simulink model "SAME5x_PIM_MCLV2_ioconfig"  (R2020b)
(part 2 of 3)

      mask TypeOptions CTXT4: Not Assigned | Alternate Register set assigned to IPL level 7 | Alternate Register set assigned to IPL level 6 | Alternate Register set assigned to IPL level 5 | Alternate Register set assigned to IPL level 4 | Alternate Register set assigned to IPL level 3 | Alternate Register set assigned to IPL level 2 | Alternate Register set assigned to IPL level 1
      mask TypeOptions MBXM0: Mailbox register configured for Master data read (Slave to Master data transfer) | Mailbox register configured for Master data write (Master to Slave data transfer)
      mask TypeOptions MBXM1: Mailbox register configured for Master data read (Slave to Master data transfer) | Mailbox register configured for Master data write (Master to Slave data transfer)
      mask TypeOptions MBXM2: Mailbox register configured for Master data read (Slave to Master data transfer) | Mailbox register configured for Master data write (Master to Slave data transfer)
      mask TypeOptions MBXM3: Mailbox register configured for Master data read (Slave to Master data transfer) | Mailbox register configured for Master data write (Master to Slave data transfer)
      mask TypeOptions MBXM4: Mailbox register configured for Master data read (Slave to Master data transfer) | Mailbox register configured for Master data write (Master to Slave data transfer)
      mask TypeOptions MBXM5: Mailbox register configured for Master data read (Slave to Master data transfer) | Mailbox register configured for Master data write (Master to Slave data transfer)
      mask TypeOptions MBXM6: Mailbox register configured for Master data read (Slave to Master data transfer) | Mailbox register configured for Master data write (Master to Slave data transfer)
      mask TypeOptions MBXM7: Mailbox register configured for Master data read (Slave to Master data transfer) | Mailbox register configured for Master data write (Master to Slave data transfer)
      mask TypeOptions MBXM8: Mailbox register configured for Master data read (Slave to Master data transfer) | Mailbox register configured for Master data write (Master to Slave data transfer)
      mask TypeOptions MBXM9: Mailbox register configured for Master data read (Slave to Master data transfer) | Mailbox register configured for Master data write (Master to Slave data transfer)
      mask TypeOptions MBXM10: Mailbox register configured for Master data read (Slave to Master data transfer) | Mailbox register configured for Master data write (Master to Slave data transfer)
      mask TypeOptions MBXM11: Mailbox register configured for Master data read (Slave to Master data transfer) | Mailbox register configured for Master data write (Master to Slave data transfer)
      mask TypeOptions MBXM12: Mailbox register configured for Master data read (Slave to Master data transfer) | Mailbox register configured for Master data write (Master to Slave data transfer)
      mask TypeOptions MBXM13: Mailbox register configured for Master data read (Slave to Master data transfer) | Mailbox register configured for Master data write (Master to Slave data transfer)
      mask TypeOptions MBXM14: Mailbox register configured for Master data read (Slave to Master data transfer) | Mailbox register configured for Master data write (Master to Slave data transfer)
      mask TypeOptions MBXM15: Mailbox register configured for Master data read (Slave to Master data transfer) | Mailbox register configured for Master data write (Master to Slave data transfer)
      mask TypeOptions MBXHSA: MSIxMBXD15 assigned to mailbox handshake protocol block A | MSIxMBXD14 assigned to mailbox handshake protocol block A | MSIxMBXD13 assigned to mailbox handshake protocol block A | MSIxMBXD12 assigned to mailbox handshake protocol block A | MSIxMBXD11 assigned to mailbox handshake protocol block A | MSIxMBXD10 assigned to mailbox handshake protocol block A | MSIxMBXD9 assigned to mailbox handshake protocol block A | MSIxMBXD8 assigned to mailbox handshake protocol block A | MSIxMBXD7 assigned to mailbox handshake protocol block A | MSIxMBXD6 assigned to mailbox handshake protocol block A | MSIxMBXD5 assigned to mailbox handshake protocol block A | MSIxMBXD4 assigned to mailbox handshake protocol block A | MSIxMBXD3 assigned to mailbox handshake protocol block A | MSIxMBXD2 assigned to mailbox handshake protocol block A | MSIxMBXD1 assigned to mailbox handshake protocol block A | MSIxMBXD0 assigned to mailbox handshake protocol block A
      mask TypeOptions MBXHSB: MSIxMBXD15 assigned to mailbox handshake protocol block B | MSIxMBXD14 assigned to mailbox handshake protocol block B | MSIxMBXD13 assigned to mailbox handshake protocol block B | MSIxMBXD12 assigned to mailbox handshake protocol block B | MSIxMBXD11 assigned to mailbox handshake protocol block B | MSIxMBXD10 assigned to mailbox handshake protocol block B | MSIxMBXD9 assigned to mailbox handshake protocol block B | MSIxMBXD8 assigned to mailbox handshake protocol block B | MSIxMBXD7 assigned to mailbox handshake protocol block B | MSIxMBXD6 assigned to mailbox handshake protocol block B | MSIxMBXD5 assigned to mailbox handshake protocol block B | MSIxMBXD4 assigned to mailbox handshake protocol block B | MSIxMBXD3 assigned to mailbox handshake protocol block B | MSIxMBXD2 assigned to mailbox handshake protocol block B | MSIxMBXD1 assigned to mailbox handshake protocol block B | MSIxMBXD0 assigned to mailbox handshake protocol block B
      mask TypeOptions MBXHSC: MSIxMBXD15 assigned to mailbox handshake protocol block C | MSIxMBXD14 assigned to mailbox handshake protocol block C | MSIxMBXD13 assigned to mailbox handshake protocol block C | MSIxMBXD12 assigned to mailbox handshake protocol block C | MSIxMBXD11 assigned to mailbox handshake protocol block C | MSIxMBXD10 assigned to mailbox handshake protocol block C | MSIxMBXD9 assigned to mailbox handshake protocol block C | MSIxMBXD8 assigned to mailbox handshake protocol block C | MSIxMBXD7 assigned to mailbox handshake protocol block C | MSIxMBXD6 assigned to mailbox handshake protocol block C | MSIxMBXD5 assigned to mailbox handshake protocol block C | MSIxMBXD4 assigned to mailbox handshake protocol block C | MSIxMBXD3 assigned to mailbox handshake protocol block C | MSIxMBXD2 assigned to mailbox handshake protocol block C | MSIxMBXD1 assigned to mailbox handshake protocol block C | MSIxMBXD0 assigned to mailbox handshake protocol block C
      mask TypeOptions MBXHSD: MSIxMBXD15 assigned to mailbox handshake protocol block D | MSIxMBXD14 assigned to mailbox handshake protocol block D | MSIxMBXD13 assigned to mailbox handshake protocol block D | MSIxMBXD12 assigned to mailbox handshake protocol block D | MSIxMBXD11 assigned to mailbox handshake protocol block D | MSIxMBXD10 assigned to mailbox handshake protocol block D | MSIxMBXD9 assigned to mailbox handshake protocol block D | MSIxMBXD8 assigned to mailbox handshake protocol block D | MSIxMBXD7 assigned to mailbox handshake protocol block D | MSIxMBXD6 assigned to mailbox handshake protocol block D | MSIxMBXD5 assigned to mailbox handshake protocol block D | MSIxMBXD4 assigned to mailbox handshake protocol block D | MSIxMBXD3 assigned to mailbox handshake protocol block D | MSIxMBXD2 assigned to mailbox handshake protocol block D | MSIxMBXD1 assigned to mailbox handshake protocol block D | MSIxMBXD0 assigned to mailbox handshake protocol block D
      mask TypeOptions MBXHSE: MSIxMBXD15 assigned to mailbox handshake protocol block E | MSIxMBXD14 assigned to mailbox handshake protocol block E | MSIxMBXD13 assigned to mailbox handshake protocol block E | MSIxMBXD12 assigned to mailbox handshake protocol block E | MSIxMBXD11 assigned to mailbox handshake protocol block E | MSIxMBXD10 assigned to mailbox handshake protocol block E | MSIxMBXD9 assigned to mailbox handshake protocol block E | MSIxMBXD8 assigned to mailbox handshake protocol block E | MSIxMBXD7 assigned to mailbox handshake protocol block E | MSIxMBXD6 assigned to mailbox handshake protocol block E | MSIxMBXD5 assigned to mailbox handshake protocol block E | MSIxMBXD4 assigned to mailbox handshake protocol block E | MSIxMBXD3 assigned to mailbox handshake protocol block E | MSIxMBXD2 assigned to mailbox handshake protocol block E | MSIxMBXD1 assigned to mailbox handshake protocol block E | MSIxMBXD0 assigned to mailbox handshake protocol block E
      mask TypeOptions MBXHSF: MSIxMBXD15 assigned to mailbox handshake protocol block F | MSIxMBXD14 assigned to mailbox handshake protocol block F | MSIxMBXD13 assigned to mailbox handshake protocol block F | MSIxMBXD12 assigned to mailbox handshake protocol block F | MSIxMBXD11 assigned to mailbox handshake protocol block F | MSIxMBXD10 assigned to mailbox handshake protocol block F | MSIxMBXD9 assigned to mailbox handshake protocol block F | MSIxMBXD8 assigned to mailbox handshake protocol block F | MSIxMBXD7 assigned to mailbox handshake protocol block F | MSIxMBXD6 assigned to mailbox handshake protocol block F | MSIxMBXD5 assigned to mailbox handshake protocol block F | MSIxMBXD4 assigned to mailbox handshake protocol block F | MSIxMBXD3 assigned to mailbox handshake protocol block F | MSIxMBXD2 assigned to mailbox handshake protocol block F | MSIxMBXD1 assigned to mailbox handshake protocol block F | MSIxMBXD0 assigned to mailbox handshake protocol block F
      mask TypeOptions MBXHSG: MSIxMBXD15 assigned to mailbox handshake protocol block G | MSIxMBXD14 assigned to mailbox handshake protocol block G | MSIxMBXD13 assigned to mailbox handshake protocol block G | MSIxMBXD12 assigned to mailbox handshake protocol block G | MSIxMBXD11 assigned to mailbox handshake protocol block G | MSIxMBXD10 assigned to mailbox handshake protocol block G | MSIxMBXD9 assigned to mailbox handshake protocol block G | MSIxMBXD8 assigned to mailbox handshake protocol block G | MSIxMBXD7 assigned to mailbox handshake protocol block G | MSIxMBXD6 assigned to mailbox handshake protocol block G | MSIxMBXD5 assigned to mailbox handshake protocol block G | MSIxMBXD4 assigned to mailbox handshake protocol block G | MSIxMBXD3 assigned to mailbox handshake protocol block G | MSIxMBXD2 assigned to mailbox handshake protocol block G | MSIxMBXD1 assigned to mailbox handshake protocol block G | MSIxMBXD0 assigned to mailbox handshake protocol block G
      mask TypeOptions MBXHSH: MSIxMBXD15 assigned to mailbox handshake protocol block H | MSIxMBXD14 assigned to mailbox handshake protocol block H | MSIxMBXD13 assigned to mailbox handshake protocol block H | MSIxMBXD12 assigned to mailbox handshake protocol block H | MSIxMBXD11 assigned to mailbox handshake protocol block H | MSIxMBXD10 assigned to mailbox handshake protocol block H | MSIxMBXD9 assigned to mailbox handshake protocol block H | MSIxMBXD8 assigned to mailbox handshake protocol block H | MSIxMBXD7 assigned to mailbox handshake protocol block H | MSIxMBXD6 assigned to mailbox handshake protocol block H | MSIxMBXD5 assigned to mailbox handshake protocol block H | MSIxMBXD4 assigned to mailbox handshake protocol block H | MSIxMBXD3 assigned to mailbox handshake protocol block H | MSIxMBXD2 assigned to mailbox handshake protocol block H | MSIxMBXD1 assigned to mailbox handshake protocol block H | MSIxMBXD0 assigned to mailbox handshake protocol block H
      mask TypeOptions HSAEN: Mailbox data flow control handshake protocol block disabled. | Mailbox data flow control handshake protocol block enabled
      mask TypeOptions HSBEN: Mailbox data flow control handshake protocol block disabled. | Mailbox data flow control handshake protocol block enabled
      mask TypeOptions HSCEN: Mailbox data flow control handshake protocol block disabled. | Mailbox data flow control handshake protocol block enabled
      mask TypeOptions HSDEN: Mailbox data flow control handshake protocol block disabled. | Mailbox data flow control handshake protocol block enabled
      mask TypeOptions HSEEN: Mailbox data flow control handshake protocol block disabled. | Mailbox data flow control handshake protocol block enabled
      mask TypeOptions HSFEN: Mailbox data flow control handshake protocol block disabled. | Mailbox data flow control handshake protocol block enabled
      mask TypeOptions HSGEN: Mailbox data flow control handshake protocol block disabled. | Mailbox data flow control handshake protocol block enabled
      mask TypeOptions HSHEN: Mailbox data flow control handshake protocol block disabled. | Mailbox data flow control handshake protocol block enabled
      mask TypeOptions CPRA0: Master core owns pin. | Slave 1 core owns pin.
      mask TypeOptions CPRA1: Master core owns pin. | Slave 1 core owns pin.
      mask TypeOptions CPRA2: Master core owns pin. | Slave 1 core owns pin.
      mask TypeOptions CPRA3: Master core owns pin. | Slave 1 core owns pin.
      mask TypeOptions CPRA4: Master core owns pin. | Slave 1 core owns pin.
      mask TypeOptions CPRB0: Master core owns pin. | Slave 1 core owns pin.
      mask TypeOptions CPRB1: Master core owns pin. | Slave 1 core owns pin.
      mask TypeOptions CPRB2: Master core owns pin. | Slave 1 core owns pin.
      mask TypeOptions CPRB3: Master core owns pin. | Slave 1 core owns pin.
      mask TypeOptions CPRB4: Master core owns pin. | Slave 1 core owns pin.
      mask TypeOptions CPRB5: Master core owns pin. | Slave 1 core owns pin.
      mask TypeOptions CPRB6: Master core owns pin. | Slave 1 core owns pin.
      mask TypeOptions CPRB7: Master core owns pin. | Slave 1 core owns pin.
      mask TypeOptions CPRB8: Master core owns pin. | Slave 1 core owns pin.
      mask TypeOptions CPRB9: Master core owns pin. | Slave 1 core owns pin.
      mask TypeOptions CPRB10: Master core owns pin. | Slave 1 core owns pin.
      mask TypeOptions CPRB11: Master core owns pin. | Slave 1 core owns pin.
      mask TypeOptions CPRB12: Master core owns pin. | Slave 1 core owns pin.
      mask TypeOptions CPRB13: Master core owns pin. | Slave 1 core owns pin.
      mask TypeOptions CPRB14: Master core owns pin. | Slave 1 core owns pin.
      mask TypeOptions CPRB15: Master core owns pin. | Slave 1 core owns pin.
      mask TypeOptions CPRC0: Master core owns pin. | Slave 1 core owns pin.
      mask TypeOptions CPRC1: Master core owns pin. | Slave 1 core owns pin.
      mask TypeOptions CPRC2: Master core owns pin. | Slave 1 core owns pin.
      mask TypeOptions CPRC3: Master core owns pin. | Slave 1 core owns pin.
      mask TypeOptions CPRC4: Master core owns pin. | Slave 1 core owns pin.
      mask TypeOptions CPRC5: Master core owns pin. | Slave 1 core owns pin.
      mask TypeOptions CPRC6: Master core owns pin. | Slave 1 core owns pin.
      mask TypeOptions CPRC7: Master core owns pin. | Slave 1 core owns pin.
      mask TypeOptions CPRC8: Master core owns pin. | Slave 1 core owns pin.
      mask TypeOptions CPRC9: Master core owns pin. | Slave 1 core owns pin.
      mask TypeOptions CPRC10: Master core owns pin. | Slave 1 core owns pin.
      mask TypeOptions CPRC11: Master core owns pin. | Slave 1 core owns pin.
      mask TypeOptions CPRC12: Master core owns pin. | Slave 1 core owns pin.
      mask TypeOptions CPRC13: Master core owns pin. | Slave 1 core owns pin.
      mask TypeOptions CPRC14: Master core owns pin. | Slave 1 core owns pin.
      mask TypeOptions CPRC15: Master core owns pin. | Slave 1 core owns pin.
      mask TypeOptions CPRD0: Master core owns pin. | Slave 1 core owns pin.
      mask TypeOptions CPRD1: Master core owns pin. | Slave 1 core owns pin.
      mask TypeOptions CPRD2: Master core owns pin. | Slave 1 core owns pin.
      mask TypeOptions CPRD3: Master core owns pin. | Slave 1 core owns pin.
      mask TypeOptions CPRD4: Master core owns pin. | Slave 1 core owns pin.
      mask TypeOptions CPRD5: Master core owns pin. | Slave 1 core owns pin.
      mask TypeOptions CPRD6: Master core owns pin. | Slave 1 core owns pin.
      mask TypeOptions CPRD7: Master core owns pin. | Slave 1 core owns pin.
      mask TypeOptions CPRD8: Master core owns pin. | Slave 1 core owns pin.
      mask TypeOptions CPRD9: Master core owns pin. | Slave 1 core owns pin.
      mask TypeOptions CPRD10: Master core owns pin. | Slave 1 core owns pin.
      mask TypeOptions CPRD11: Master core owns pin. | Slave 1 core owns pin.
      mask TypeOptions CPRD12: Master core owns pin. | Slave 1 core owns pin.
      mask TypeOptions CPRD13: Master core owns pin. | Slave 1 core owns pin.
      mask TypeOptions CPRD14: Master core owns pin. | Slave 1 core owns pin.
      mask TypeOptions CPRD15: Master core owns pin. | Slave 1 core owns pin.
      mask TypeOptions CPRE0: Master core owns pin. | Slave 1 core owns pin.
      mask TypeOptions CPRE1: Master core owns pin. | Slave 1 core owns pin.
      mask TypeOptions CPRE2: Master core owns pin. | Slave 1 core owns pin.
      mask TypeOptions CPRE3: Master core owns pin. | Slave 1 core owns pin.
      mask TypeOptions CPRE4: Master core owns pin. | Slave 1 core owns pin.
      mask TypeOptions CPRE5: Master core owns pin. | Slave 1 core owns pin.
      mask TypeOptions CPRE6: Master core owns pin. | Slave 1 core owns pin.
      mask TypeOptions CPRE7: Master core owns pin. | Slave 1 core owns pin.
      mask TypeOptions CPRE8: Master core owns pin. | Slave 1 core owns pin.
      mask TypeOptions CPRE9: Master core owns pin. | Slave 1 core owns pin.
      mask TypeOptions CPRE10: Master core owns pin. | Slave 1 core owns pin.
      mask TypeOptions CPRE11: Master core owns pin. | Slave 1 core owns pin.
      mask TypeOptions CPRE12: Master core owns pin. | Slave 1 core owns pin.
      mask TypeOptions CPRE13: Master core owns pin. | Slave 1 core owns pin.
      mask TypeOptions CPRE14: Master core owns pin. | Slave 1 core owns pin.
      mask TypeOptions CPRE15: Master core owns pin. | Slave 1 core owns pin.
      mask TypeOptions S1FNOSC: Internal Fast RC (FRC) Oscillator with postscaler | Back up Fast RC (BFRC) Oscillator | Low-Power RC Oscillator (LPRC) | Primary Oscillator with PLL module (XT + PLL; HS + PLL; EC + PLL) | Primary Oscillator (XT; HS; EC) | Fast RC Oscillator with divide-by-N with PLL module (FRCPLL)  | Internal Fast RC (FRC)
      mask TypeOptions S1IESO: Start up with FRC; then switch | Disable
      mask TypeOptions S1OSCIOFNC: OSC2 is clock output | general purpose digital I/O pin
      mask TypeOptions S1FCKSM: Both Clock switching and Fail-safe Clock Monitor are disabled | Clock switching is enabled;Fail-safe Clock Monitor is disabled | Both Clock switching and Fail-safe Clock Monitor are enabled
      mask TypeOptions S1PLLKEN: S1PLLKEN_ON | S1PLLKEN_OFF
      mask TypeOptions S1RWDTPS: 1:1048576 | 1:524288 | 1:262144 | 1:131072 | 1:65536 | 1:32768 | 1:16384 | 1:8192 | 1:4096 | 1:2048 | 1:1024 | 1:512 | 1:256 | 1:128 | 1:64 | 1:32 | 1:16 | 1:8 | 1:4 | 1:2 | 1:1
      mask TypeOptions S1RCLKSEL: Always use LPRC | Use FRC when WINDIS = 0; system clock is not INTOSC/LPRC and device is not in Sleep; otherwise; use INTOSC/LPRC | Use peripheral clk when system clock is not INTOSC/LPRC and device is not in Sleep;otherwise; use INTOSC/LPRC
      mask TypeOptions S1WINDIS: Watchdog Timer operates in Non-Window mode | Watchdog Timer operates in Window mode
      mask TypeOptions S1WDTWIN: WDT Window is 25% of WDT period | WDT Window is 37.5% of WDT period | WDT Window is 50% of WDT period | WDT Windo is 75% of WDT period
      mask TypeOptions S1SWDTPS: 1:1048576 | 1:524288 | 1:262144 | 1:131072 | 1:65536 | 1:32768 | 1:16384 | 1:8192 | 1:4096 | 1:2048 | 1:1024 | 1:512 | 1:256 | 1:128 | 1:64 | 1:32 | 1:16 | 1:8 | 1:4 | 1:2 | 1:1
      mask TypeOptions S1FWDTEN: Enable | Disable
      mask TypeOptions S1ICS: Communicate on PGC1 and PGD1 | Communicate on PGC2 and PGD2 | Communicate on PGC3 and PGD3
      mask TypeOptions S1DEBUG: Not used
      mask TypeOptions S1ISOLAT: The slave can operate (in debug mode) even if the SLVEN bit in the MSI is zero. | The slave can only operate if the SLVEN bit in the MSI is set.
      mask TypeOptions S1NOBTSWP: BOOTSWP instruction is disabled | BOOTSWP instruction is enabled
      mask TypeOptions S1ALTI2C1: I2C1 mapped to SDA1/SCL1 pins | I2C1 mapped to ASDA1/ASCL1 pins
      mask TypeOptions S1SPI1PIN: Slave SPI1 uses I/O remap (PPS) pins | Slave SPI1 uses dedicated I/O pins
      mask TypeOptions S1SSRE: Slave generated resets will reset the Slave Enable Bit in the MSI module | Slave generated resets will not reset the Slave Enable Bit in the MSI module
      mask TypeOptions S1MSRE: The master software oriented RESET events (RESET Op-Code; Watchdog timeout; TRAP reset; illegalInstruction) will also cause the slave subsystem to reset. | The master software oriented RESET events (RESET Op-Code; Watchdog timeout; TRAP reset; illegalInstruction) will not cause the slave subsystem to reset.
      mask TypeOptions S1CTXT1: Not Assigned | Alternate Register set assigned to IPL level 7 | Alternate Register set assigned to IPL level 6 | Alternate Register set assigned to IPL level 5 | Alternate Register set assigned to IPL level 4 | Alternate Register set assigned to IPL level 3 | Alternate Register set assigned to IPL level 2 | Alternate Register set assigned to IPL level 1
      mask TypeOptions S1CTXT2: Not Assigned | Alternate Register set assigned to IPL level 7 | Alternate Register set assigned to IPL level 6 | Alternate Register set assigned to IPL level 5 | Alternate Register set assigned to IPL level 4 | Alternate Register set assigned to IPL level 3 | Alternate Register set assigned to IPL level 2 | Alternate Register set assigned to IPL level 1
      mask TypeOptions S1CTXT3: Not Assigned | Alternate Register set assigned to IPL level 7 | Alternate Register set assigned to IPL level 6 | Alternate Register set assigned to IPL level 5 | Alternate Register set assigned to IPL level 4 | Alternate Register set assigned to IPL level 3 | Alternate Register set assigned to IPL level 2 | Alternate Register set assigned to IPL level 1
      mask TypeOptions S1CTXT4: Not Assigned | Alternate Register set assigned to IPL level 7 | Alternate Register set assigned to IPL level 6 | Alternate Register set assigned to IPL level 5 | Alternate Register set assigned to IPL level 4 | Alternate Register set assigned to IPL level 3 | Alternate Register set assigned to IPL level 2 | Alternate Register set assigned to IPL level 1
      mask TypeOptions BORLVL: Not used
      mask TypeOptions BSSO: Not used
      mask TypeOptions MCA: Not used
      mask TypeOptions MAXTEMP: Not used
      mask TypeOptions CFGAN14: Not used
      mask TypeOptions CFGAN15: Not used
      mask TypeOptions S1IOL1WAY: Not used
      mask TypeOptions S1BSSO: Not used
      mask TypeOptions S1BACKBUG: Not used
      mask TypeOptions BISTDIS: mBIST on reset feature disabled | mBIST on reset feature enabled
      mask TypeOptions NOBTSWP: BOOTSWP instruction is disabled | BOOTSWP instruction is enabled
      mask TypeOptions S1BISTDIS: Slave BIST on reset feature disabled | Slave BIST on reset feature enabled
      mask TypeOptions S1DMTIVTL: Not used
      mask TypeOptions S1DMTIVTH: Not used
      mask TypeOptions S1DMTCNTL: Not used
      mask TypeOptions S1DMTCNTH: Not used
      mask TypeOptions S1DMTDIS: Slave Dead Man Timer is Disabled and can be enabled by software | Slave Dead Man Timer is Enabled and cannot be disabled by software
      mask TypeOptions BSEQ: Not used
      mask TypeOptions IBSEQ: Not used
      mask TypeOptions SMB3EN: SMBus 3.0 input levels | Normal  SMBus input levels
      mask TypeOptions FUSBIDIO2: USBID pin is controlled by the USB2 module | USBID pin is controlled by the port function
      mask TypeOptions FVBUSIO2: VBUSON pin is controlled by the USB2 module | VBUSON pin is controlled by the port function
      mask TypeOptions FUSBIDIO1: USBID pin is controlled by the USB1 module | USBID pin is controlled by the port function
      mask TypeOptions FVBUSIO1: VBUSON pin is controlled by the USB1 module | VBUSON pin is controlled by the port function
      mask TypeOptions VBATBOREN: Enable ZPBOR during VBAT Mode | Disable ZPBOR during VBAT Mode
      mask TypeOptions FDSEN: Enable DSEN bit in DSCON | Disable DSEN bit in DSCON
      mask TypeOptions BORSEL: BOR trip voltage 2.1v (Non-OPAMP deviced operation) | BOR trip voltage 2.8v (OPAMP deviced operation)
      mask TypeOptions POSCFGAIN: Gain is G3 | Gain is G2 | Gain is G1 | Gain is G0
      mask TypeOptions POSCAGCDLY: Settling time = 25ms x AGCRNG | Settling time = 6.25ms x AGCRNG | Settling time = 400ms x AGCRNG | Settling time = 100ms x AGCRNG
      mask TypeOptions POSCAGCRNG: Range 1x | Range 5x
      mask TypeOptions POSCAGC: Automatic Gain Control for Oscillator | Manual Gain Control of Oscillator
      mask TypeOptions FDBGWP: Not used
      mask DialogControl ParameterTabVar0 Prompt: General
      mask DialogControl ParameterTabVar01 Prompt: Oscillator
      mask DialogControl ParameterTabVar012 Prompt: Memory
      mask DialogControl ParameterTabVar0123 Prompt: Debug
      mask DialogControl ParameterTabVar01234 Prompt: DualCore
      mask Display: MCHP_DrawLogo;fprintf('MCHP_MASTER\\nSAME54P20A - TQFP128\\n100MHZ');
  Model Info : simulink/Model-Wide Utilities/Model Info  Frame=on  DisplayStringWithTags=|  HorizontalTextAlignment=Center  LeftAlignmentValue=0.5
      | %<ModelName> v%<ModelVersion> - %<Creator>
      | 
      | %<Description>
      | 
      | Last modified on: %<LastModificationDate>
  PWM : Subsystem
  Port Info : S-Function  FunctionName=MCHP_EmptySFunction  SFunctionDeploymentMode=off  EnableBusSupport=off  mask{MCHP_MASTERLINK=SAME5x_PIM_MCLV2_ioconfig/Microchip Master}
      mask init:
      | MCHP_PortInfo_Callback(gcbh,'INITIALISATION');
      settings: CopyFcn=MCHP_PortInfo_Callback(gcb,'COPY');  OpenFcn=MCHP_PortInfo_Callback(gcb,'OPEN');
      mask Display: MCHP_DrawLogo;text(.05,20,'[Pin]  Port   -  Desc\n [23]   PA6  -  ADC0_AIN6 -  ( ADC0_AIN1 )\n [33]   PA8  -  TCC0_WO0 -  ( PWM0_H0 )\n [34]   PA9  -  TCC0_WO1 -  ( PWM0_H1 )\n [35]   PA10 -  TCC0_WO2 -  ( PWM0_H2 )\n [48]   PD9  -  DIN -  ( Digital In )\n [60]   PA12 -  SERCOM2_PAD0 -  ( UART2 Tx )\n [61]   PA13 -  SERCOM2_PAD1 -  ( UART2 Rx )\n [66]   PA16 -  TCC0_WO4 -  ( PWM0_L0 )\n [67]   PA17 -  TCC0_WO5 -  ( PWM0_L1 )\n [68]   PA18 -  TCC0_WO6 -  ( PWM0_L2 )\n [70]   PC16 -  PDEC_QDI0 -  ( PDEC A )\n [71]   PC17 -  PDEC_QDI1 -  ( PDEC B )\n [72]   PC18 -  PDEC_QDI2 -  ( PDEC index )\n[102]   PB26 -  DOU -  ( Digital Out )','verticalalignment','Top','horizontalalignment','left');text(.95,0.05,'(14 pins)','verticalalignment','Bottom','horizontalalignment','right');
  Rate Transition{1..5} (5 alike) : RateTransition
  Selecteur : Subsystem
  Subsystem : Subsystem
  UART Configuration : S-Function  InitFcn=MCHP_UART_Config_Callback(gcbh,'InitFcn');  FunctionName=MCHP_UART_Config  SFunctionDeploymentMode=off  EnableBusSupport=off  mask(Configuration for UART peripheral){UART_REF=SERCOM USART 2, BAUD_Choice=Dynamic Options, BAUD_Choice_TXT=115200         [-0.00%], BAUD_Choice_IR=Dynamic Options, BAUD_Choice_IR_TXT=[], BAUD_Custom=1000000, INT_PRIORITY=3, ALT_IO=on, PIN_RX=Dynamic Options, PIN_RX_TXT=PA13 / Pin[61] / pad1, PIN_TX=Dynamic Options, PIN_TX_TXT=PA12 / Pin[60] / pad0, MCHP_PORT={UART2 Rx}{SERCOM2_PAD1}3:0:P13;{UART2 Tx}{SERCOM2_PAD0}3:1:P12;, MCHP_MASTERLINK=SAME5x_PIM_MCLV2_ioconfig/Microchip Master, MCHP_COM_ExtPil=off, TX_IMPLEMENTATION=Circular Buffer, TX_IMPLEMENTATION_default=Circular Buffer, TX_INT_PRIORITY=4, TX_INT_WHEN=is empty, TX_INT_WHEN_default=is empty & last char is sent, TX_CIRCULAR_SIZE=512, TX_DMA_CHANNEL=0, TX_DMA_SIZE=[], TX_TASK_PROTECTION=Delay tasks (default), TX_INTERRUPT_PROTECTION=Do not send on conflict (default), TX_INTERRUPT_PROTECTION_default=Do not send on conflict (default), RX_IMPLEMENTATION=Circular Buffer, RX_IMPLEMENTATION_default=Circular Buffer, RX_INT_PRIORITY=4, RX_INT_WHEN=receive 1 character, RX_CIRCULAR_SIZE=512, RX_DMA_CHANNEL=0, RX_DMA_SIZE=0, DuplexMode=Full duplex (default), PIN_RX_Inv=off, PIN_TX_Inv=off, PIN_RXTX_Inv=off, ParityBit=No parity (default), StopBit=1 stop bit (default), IRDA=off, FlowControl=None, PIN_CTS=Dynamic Options, PIN_CTS_TXT=PA10 / Pin[35] / pad2, PIN_RTS=Dynamic Options, PIN_RTS_TXT=PA11 / Pin[36] / pad3, InitSequence_chkbox=off, BAUD_Choice_InitSeq=Dynamic Options, BAUD_Choice_InitSeq_TXT=115200         [-0.00%], BAUD_Choice_IR_InitSeq=Dynamic Options, BAUD_Choice_IR_InitSeq_TXT=0, BAUD_Custom_InitSeq=0, InitSequence='Hello World'}
      mask prompts: UART_REF "Ref UART"; BAUD_Choice "Current Baud: [ 115204 ]"; BAUD_Choice_TXT "Baud_Choixe_TXT"; BAUD_Choice_IR "Current Baud: [ 115204 ]"; BAUD_Custom "Custom Baud: 109306 with -5.12% Error"; INT_PRIORITY "Interrupt Priority [ Rx Tx ]"; ALT_IO "Alternative I/O"; PIN_RX "Rx Pin"; PIN_TX "Tx Pin"; TX_IMPLEMENTATION "Implementation"; TX_IMPLEMENTATION_default "Implementation"; TX_INT_PRIORITY "Interrupt Priority"; TX_INT_WHEN "Interrupt when Transmit Buffer"; TX_INT_WHEN_default "Interrupt when Transmit Buffer"; TX_CIRCULAR_SIZE "Circular Buffer size"; TX_DMA_CHANNEL "DMA Channel"; TX_DMA_SIZE "DMA Buffer size"; TX_TASK_PROTECTION "Task intertwined Tx protection"; TX_INTERRUPT_PROTECTION "Asynchronous intertwined Tx protection"; TX_INTERRUPT_PROTECTION_default "Asynchronous intertwined Tx protection"; RX_IMPLEMENTATION "Implementation"; RX_IMPLEMENTATION_default "Implementation"; RX_INT_PRIORITY "Interrupt Priority"; RX_INT_WHEN "Interrupt when Receive Buffer"; RX_CIRCULAR_SIZE "Circular Buffer size"; RX_DMA_CHANNEL "DMA Channel"; RX_DMA_SIZE "DMA Buffer size"; DuplexMode "Duplex"; PIN_RX_Inv "Invert Rx Pin logic (Idle state is low level)"; PIN_TX_Inv "Invert Tx Pin logic (Idle state is low level)"; PIN_RXTX_Inv "Invert Rx & Tx Pin logic (Idle state is low level)"; ParityBit "Parity"; StopBit "Stop bit"; IRDA "IrDA Mode"; FlowControl "Hardware Flow Control"; PIN_CTS "CTS Pin (input)"; PIN_RTS "RTS Pin (output)"; InitSequence_chkbox "Send an Initialisation sequence on the UART"; BAUD_Choice_InitSeq "Current Baud: [ 115204 ]"; BAUD_Choice_InitSeq_TXT "Baud_Choixe_TXT"; BAUD_Choice_IR_InitSeq "Current Baud: [ 115204 ]"; BAUD_Choice_IR_InitSeq_TXT "Baud_Choice_IR_TXT"; BAUD_Custom_InitSeq "Custom Baud: 109306 with -5.12% Error"; InitSequence "Initialisaiton sequence to send (String or vector)"
      mask help: Configure UART parameters.
      mask init:
      | MCHP_UART_Config_Callback(gcbh,'INITIALISATION');
      settings: CopyFcn=MCHP_UART_Config_Callback(gcbh,'CopyFcn');  PreSaveFcn=MCHP_Fun.PreSaveFcn_DynamicOptions(gcbh);  OpenFcn=MCHP_UART_Config_Callback(gcbh,'OPEN');
      mask TypeOptions UART_REF: SERCOM USART 0 | SERCOM USART 1 | SERCOM USART 2 | SERCOM USART 3 | SERCOM USART 4 | SERCOM USART 5 | SERCOM USART 6 | SERCOM USART 7
      mask Callback UART_REF: MCHP_UART_Config_Callback(gcbh,'UART_REF');
      mask TypeOptions BAUD_Choice: Dynamic Options
      mask Callback BAUD_Choice: MCHP_UART_Config_Callback(gcbh,'BAUD_Choice');
      mask TypeOptions BAUD_Choice_IR: Dynamic Options
      mask Callback BAUD_Choice_IR: MCHP_UART_Config_Callback(gcbh,'BAUD_Choice_IR');
      mask Callback BAUD_Choice_IR_TXT: % This field is not used
      mask Callback BAUD_Custom: MCHP_UART_Config_Callback(gcbh,'BAUD_Custom');
      mask TypeOptions INT_PRIORITY: 0 | 1 | 2 | 3 | 4 | 5 | 6 | 7
      mask TypeOptions PIN_RX: Dynamic Options
      mask TypeOptions PIN_TX: Dynamic Options
      mask TypeOptions TX_IMPLEMENTATION: Do not implement Tx | Simplest (1 bytes internal buffer only) | Circular Buffer
      mask Callback TX_IMPLEMENTATION: MCHP_UART_Config_Callback(gcbh,'TX_IMPLEMENTATION');
      mask TypeOptions TX_IMPLEMENTATION_default: Circular Buffer
      mask TypeOptions TX_INT_PRIORITY: 0 | 1 | 2 | 3 | 4 | 5 | 6 | 7
      mask TypeOptions TX_INT_WHEN: is empty | is empty & last char is sent | has one empty space
      mask TypeOptions TX_INT_WHEN_default: is empty & last char is sent
      mask TypeOptions TX_CIRCULAR_SIZE: 4 | 8 | 16 | 32 | 64 | 128 | 256 | 512 | 1024 | 2048 | 4096 | 8192 | 16384 | 32768
      mask TypeOptions TX_DMA_CHANNEL: 0  | 1 | 2 | 3 | 4 | 5 | 6 | 7 | 8 | 9 | 10  | 11 | 12 | 13 | 14 | 15 | 16 | 17 | 18 | 19 | 20  | 21 | 22 | 23
      mask TypeOptions TX_TASK_PROTECTION: Delay tasks (default) | Do not send on conflict | no protection
      mask Callback TX_TASK_PROTECTION: MCHP_UART_Config_Callback(gcbh,'TX_TASK_PROTECTION');
      mask TypeOptions TX_INTERRUPT_PROTECTION: Do not send on conflict (default) | Delay all interrupts | no protection
      mask TypeOptions TX_INTERRUPT_PROTECTION_default: Do not send on conflict (default)
      mask TypeOptions RX_IMPLEMENTATION: Do not implement Rx | Simplest (1 bytes internal buffer only) | Circular Buffer
      mask Callback RX_IMPLEMENTATION: MCHP_UART_Config_Callback(gcbh,'RX_IMPLEMENTATION');
      mask TypeOptions RX_IMPLEMENTATION_default: Circular Buffer
      mask TypeOptions RX_INT_PRIORITY: 1 | 2 | 3 | 4 | 5 | 6 | 7
      mask TypeOptions RX_INT_WHEN: is full (contains 4 data characters) | is 3/4 fulll (contains 3 data characters) | receive 1 character
      mask TypeOptions RX_CIRCULAR_SIZE: 4 | 8 | 16 | 32 | 64 | 128 | 256 | 512 | 1024 | 2048 | 4096 | 8192 | 16384 | 32768
      mask TypeOptions RX_DMA_CHANNEL: 0  | 1 | 2 | 3 | 4 | 5 | 6 | 7 | 8 | 9 | 10  | 11 | 12 | 13 | 14 | 15 | 16 | 17 | 18 | 19 | 20  | 21 | 22 | 23
      mask TypeOptions DuplexMode: Full duplex (default) | Half duplex for one wire Rx-Tx specific case
      mask Callback DuplexMode: MCHP_UART_Config_Callback(gcbh,'DuplexMode');
      mask TypeOptions ParityBit: No parity (default) | Even | Odd
      mask TypeOptions StopBit: 1 stop bit (default) | 2 stop bits
      mask Callback IRDA: MCHP_UART_Config_Callback(gcbh,'IRDA');
      mask TypeOptions FlowControl: None | RTS / CTS
      mask Callback FlowControl: MCHP_UART_Config_Callback(gcbh,'FlowControl');
      mask TypeOptions PIN_CTS: Dynamic Options
      mask TypeOptions PIN_RTS: Dynamic Options
      mask Callback InitSequence_chkbox: MCHP_UART_Config_Callback(gcbh,'InitSequence_chkbox');
      mask TypeOptions BAUD_Choice_InitSeq: Dynamic Options
      mask Callback BAUD_Choice_InitSeq: MCHP_UART_Config_Callback(gcbh,'BAUD_Choice_InitSeq');
      mask TypeOptions BAUD_Choice_IR_InitSeq: Dynamic Options
      mask Callback BAUD_Choice_IR_InitSeq: MCHP_UART_Config_Callback(gcbh,'BAUD_Choice_IR_InitSeq');
      mask Callback BAUD_Custom_InitSeq: MCHP_UART_Config_Callback(gcbh,'BAUD_Custom_InitSeq');
      mask DialogControl ParameterTabVar0 Prompt: Main
      mask DialogControl ParameterTabVar01 Prompt: Tx
      mask DialogControl ParameterTabVar012 Prompt: Rx
      mask DialogControl ParameterTabVar0123 Prompt: Advanced
      mask DialogControl ParameterTabVar01234 Prompt: Initialisation Sequence
      mask Display: MCHP_DrawLogo;fprintf('SERCOM UART 2 Config\n%u (%+5.2f%%)\nBytes / Step: %5.2f',115200,-0.0033485,0.57602);
  UART Tx-Matlab1 : MCHP_Blockset/BUS UART/UART Tx-Matlab  UART_REF=2  CHANNELS=[1:4]  AllOrNothing=off  SampleTime=0.001  MCHP_MASTERLINK=SAME5x_PIM_MCLV2_ioconfig/Microchip Master  MCHP_COMPILED_INFO="CompiledSampleTime= [0.0010000000000000000208   0 ];CompiledInportDataTypes=[  5   5   5   5 ];CompiledInportDataWidth=[1  1  1  1];"
      settings: SourceProductName=MPLAB Device Blocks for Simulink
  picgui Graphical interface : MCHP_Blockset/BUS UART/picgui Graphical interface  Nothing=0
      settings: SourceProductName=MPLAB Device Blocks for Simulink
  wires:
  Data Type Conversion/1 -> DBG_LED2/1
  Counter Limited/1 -> Data Type Conversion/1  "U2 CH1"
  Rate Transition1/1 -> UART Tx-Matlab1/2  "U2 CH2"
  Subsystem/1(U2 CH2) -> Rate Transition1/1
  Selecteur/1(Mode) -> Commande/1(commande), [mode], Rate Transition2/1
  PWM/1(PWM [0 1]) -> Subsystem/2(PWM [0 1])
  Rate Transition2/1 -> Subsystem/1(mode)
  Inv Park/1(vabc) -> PWM/1(vabc)
  Rate Transition3/1 -> UART Tx-Matlab1/1  "U2 CH1"
  [mode] -> Rate Transition3/1
  Subsystem/2(cos(pth)sin(pth)) -> Inv Park/1(cossin)
  Commande/1(vdq) -> Inv Park/2(vdq)
  Rate Transition4/1 -> UART Tx-Matlab1/3  "U2 CH3"
  Rate Transition5/1 -> UART Tx-Matlab1/4  "U2 CH4"
